simulink model "dve_nadrze_nelinear"  (R2020a)
settings: Solver=VariableStepAuto  StartTime=0.0  StopTime=t  RelTol=1e-3
values from neighbouring files (symbols this model uses):
  c2 = cp    (= 0.6)    [control_file.m]
  cp = 0.6    [control_file.m]
  dQ = 0*U    (= 0)    [control_file.m]
  g = 10    [control_file.m]
  h1condition = 0    [control_file.m]
  h2condition = 0    [control_file.m]
  S = 25e-4    (= 0.0025)    [control_file.m]
  S2 = S2_1    [control_file.m]
  Sp = Sp_1    [control_file.m]
  stepTime = t/4    (= 500)    [control_file.m]
  U = 1.2*i    [control_file.m]
settings Model: Creator=Filip Jašek  LastModifiedBy=Filip Jašek

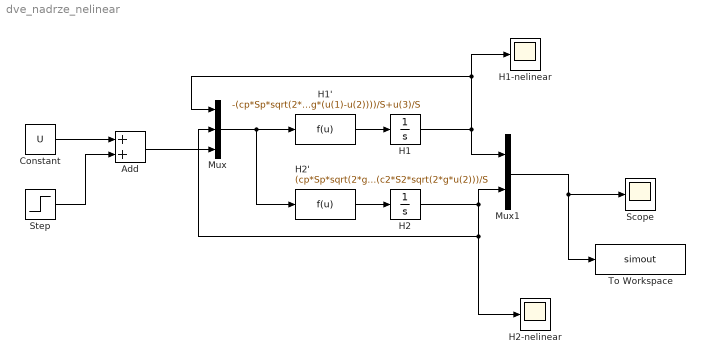
== system dve_nadrze_nelinear ==
  Add : Sum
  Constant : Constant  Value=U
  H1 : Integrator  InitialCondition=h1condition
  H1' : Fcn  Expr=-(cp*Sp*sqrt(2*g*(u(1)-u(2))))/S+u(3)/S
  H1-nelinear : Scope
  H2 : Integrator  InitialCondition=h2condition
  H2' : Fcn  Expr=(cp*Sp*sqrt(2*g*(u(1)-u(2))))/S-(c2*S2*sqrt(2*g*u(2)))/S
  H2-nelinear : Scope
  Mux : Mux  Inputs=3
  Mux1 : Mux  Inputs=2
  Scope : Scope
  Step : Step  Time=stepTime  After=dQ  SampleTime=0
  To Workspace : ToWorkspace  VariableName=simout  SaveFormat=Timeseries  SampleTime=-1
  wires:
  Mux/1 -> H2'/1, H1'/1
  H2/1 -> H2-nelinear/1, Mux/2, Mux1/2
  Mux1/1 -> To Workspace/1, Scope/1
  H2'/1 -> H2/1
  H1/1 -> H1-nelinear/1, Mux/1, Mux1/1
  H1'/1 -> H1/1
  Constant/1 -> Add/1
  Add/1 -> Mux/3
  Step/1 -> Add/2
